simulink model "NRZ"  (R2020a)
settings: Solver=VariableStepAuto  StartTime=0.0  StopTime=10.0  RelTol=1e-3
libraries: simulink x1, commrandsrc3 x1
settings Model: Creator=Rohit  LastModifiedBy=Rohit

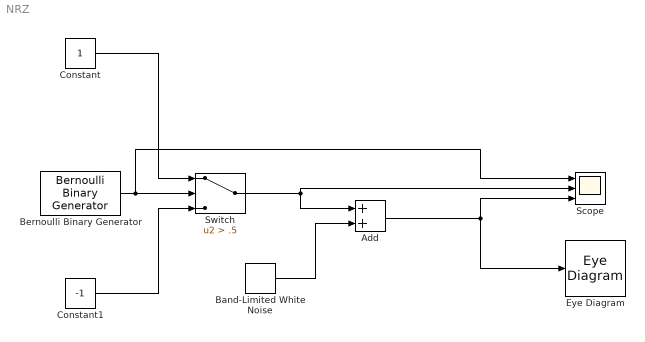
== system NRZ ==
  Add : Sum
  Band-Limited White Noise : simulink/Sources/Band-Limited White Noise  Cov=[0.0001]  Ts=0.1  seed=[23341]
  Bernoulli Binary Generator : commrandsrc3/Bernoulli Binary Generator  ProbabilityOfZero=0.5  SeedSource=Auto  Seed=0  SampleTime=1  SamplesPerFrame=1  OutputDataType=double  SimulateUsing=Interpreted execution
  Constant : Constant
  Constant1 : Constant  Value=-1
  Eye Diagram : EyeDiagram
  Scope : Scope  NumInputPorts=3
  Switch : Switch  Criteria=u2 > Threshold  Threshold=.5
  wires:
  Bernoulli Binary Generator/1 -> Scope/1, Switch/2
  Constant1/1 -> Switch/3
  Constant/1 -> Switch/1
  Band-Limited White Noise/1 -> Add/2
  Switch/1 -> Scope/2, Add/1
  Add/1 -> Eye Diagram/1, Scope/3
